simulink model "model"  (R2014b)
settings: Solver=ode45  StartTime=0.0  StopTime=10.0  RelTol=1e-3
values from neighbouring files (symbols this model uses):
  a0 = 6    [fzad2.m]    (also in zad1.m; zad2.m; zad3.m)
  a1 = 4    [fzad2.m]    (also in zad1.m; zad2.m; zad3.m)
  a2 = 3    [fzad2.m]    (also in zad1.m; zad2.m; zad3.m)
  b = 3    [fzad2.m]    (also in zad1.m; zad2.m; zad3.m)
  K = wektor(1)    [fzad2.m]    (also in zad1.m = 1; zad2.m = optymalne(1); zad3.m = 1.2)
  Ki = 1    [fzad2.m]    (also in zad1.m; zad2.m; zad3.m)
  Td = wektor(3)    [fzad2.m]    (also in zad1.m = 0; zad2.m = optymalne(3); zad3.m = 0.3975)
  Ti = wektor(2)    [fzad2.m]    (also in zad1.m = 6; zad2.m = optymalne(2); zad3.m = 1.59)
  zadana = 25    [fzad2.m]    (also in zad1.m; zad2.m; zad3.m = 1)
settings Model: Creator=Dyzio  LastModifiedBy=Dyzio

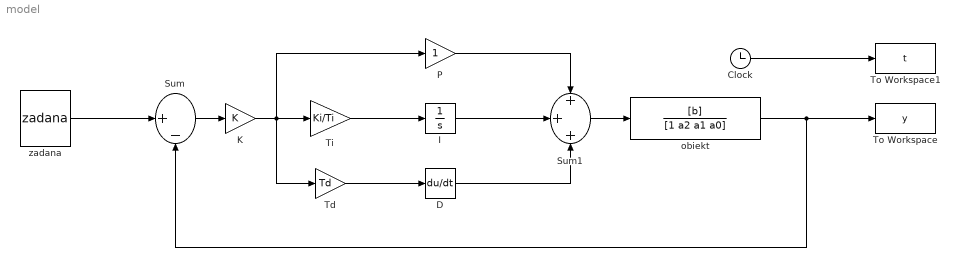
== system model ==
  Clock : Clock
  D : Derivative
  I : Integrator
  K : Gain  Gain=K
  P : Gain
  Sum : Sum  Inputs=|+-
  Sum1 : Sum  Inputs=+++
  Td : Gain  Gain=Td
  Ti : Gain  Gain=Ki/Ti
  To Workspace : ToWorkspace  VariableName=y  SampleTime=-1
  To Workspace1 : ToWorkspace  VariableName=t  SampleTime=-1
  obiekt : TransferFcn  Numerator=[b]  Denominator=[1 a2 a1 a0]
  zadana : Constant  Value=zadana
  wires:
  zadana/1 -> Sum/1
  Sum/1 -> K/1
  P/1 -> Sum1/1
  K/1 -> Td/1, Ti/1, P/1
  Ti/1 -> I/1
  I/1 -> Sum1/2
  Sum1/1 -> obiekt/1
  Td/1 -> D/1
  D/1 -> Sum1/3
  obiekt/1 -> Sum/2, To Workspace/1
  Clock/1 -> To Workspace1/1
